simulink model "pfbtest"  (R2015a)
settings: Solver=ode45  StartTime=0.0  StopTime=1500  RelTol=1e-3
libraries: xbsIndex_r4 x275
(part 1 of 2)
settings Model: Creator=tmadden  LastModifiedBy=tmadden
settings OptimizationCC: ExpressionDepthLimit=2147483647
settings DebuggingCC: UnderspecifiedInitializationDetection=Classic  MergeDetectMultiDrivingBlocksExec=none  SolverPrmCheckMsg=warning  StateNameClashWarn=warning

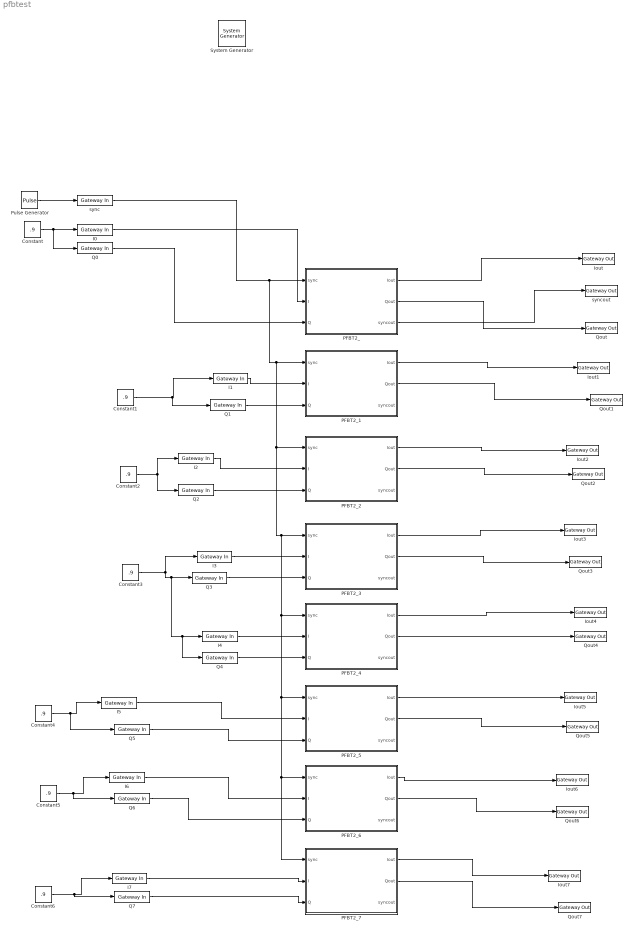
== system pfbtest ==
  " System Generator" : xbsIndex_r4/ System Generator  Tag=genX  xilinxfamily=zynq  part=xc7z100  speed=-2  package=ffv900  synthesis_tool=XST  clock_wrapper=Clock Enables  directory=./untitled/sysgen  proj_type=Project Navigator  Synth_file=XST Defaults  Impl_file=ISE Defaults  testbench=off  simulink_period=1  sysclk_period=10  dcm_input_clock_period=10  incr_netlist=off  trim_vbits=Everywhere in SubSystem  dbl_ovrd=According to Block Masks  core_generation=According to Block Masks  run_coregen=off  deprecated_control=off  eval_field=0  block_type=sysgen
  Constant{,1..6} (7 alike) : Constant  Value=.9
  I{0..7} (8 alike) : xbsIndex_r4/Gateway In  gui_display_data_type=Fixed-point  arith_type="Signed  (2's comp)"  n_bits=18  bin_pt=16  preci_type=Single  exp_width=8  frac_width=24  rows=1  columns=1  quantization="Round  (unbiased: +/- Inf)"  overflow=Saturate  period=1  UseAsADC=off  ADCChannel='1'  interface=None  automatic_assignment=on  address_offset=hex2dec('00')  intf_name=''  intf_description=''  timing_constraint=None  locs_specified=off  LOCs={}  io_standard={}  inherit_from_input=off  hdl_port=on  dbl_ovrd=off  block_type=gatewayin
  Iout{,1..7} (8 alike) : xbsIndex_r4/Gateway Out  inherit_from_input=off  hdl_port=on  rows=1  columns=1  UseAsDAC=off  DACChannel='1'  interface=None  automatic_assignment=on  address_offset=hex2dec('00')  intf_name=''  intf_description=''  timing_constraint=None  locs_specified=off  LOCs={}  io_standard={}  block_type=gatewayout
  PFBT2_ : Subsystem
  PFBT2_1 : Subsystem
  PFBT2_2 : Subsystem
  PFBT2_3 : Subsystem
  PFBT2_4 : Subsystem
  PFBT2_5 : Subsystem
  PFBT2_6 : Subsystem
  PFBT2_7 : Subsystem
  Pulse Generator : DiscretePulseGenerator  Period=1024
  Q{0..7} (8 alike) : xbsIndex_r4/Gateway In  gui_display_data_type=Fixed-point  arith_type="Signed  (2's comp)"  n_bits=18  bin_pt=16  preci_type=Single  exp_width=8  frac_width=24  rows=1  columns=1  quantization="Round  (unbiased: +/- Inf)"  overflow=Saturate  period=1  UseAsADC=off  ADCChannel='1'  interface=None  automatic_assignment=on  address_offset=hex2dec('00')  intf_name=''  intf_description=''  timing_constraint=None  locs_specified=off  LOCs={}  io_standard={}  inherit_from_input=off  hdl_port=on  dbl_ovrd=off  block_type=gatewayin
  Qout{,1..7} (8 alike) : xbsIndex_r4/Gateway Out  inherit_from_input=off  hdl_port=on  rows=1  columns=1  UseAsDAC=off  DACChannel='1'  interface=None  automatic_assignment=on  address_offset=hex2dec('00')  intf_name=''  intf_description=''  timing_constraint=None  locs_specified=off  LOCs={}  io_standard={}  block_type=gatewayout
  sync : xbsIndex_r4/Gateway In  gui_display_data_type=Boolean  arith_type=Boolean  n_bits=16  bin_pt=14  preci_type=Single  exp_width=8  frac_width=24  rows=1  columns=1  quantization="Round  (unbiased: +/- Inf)"  overflow=Saturate  period=1  UseAsADC=off  ADCChannel='1'  interface=None  automatic_assignment=on  address_offset=hex2dec('00')  intf_name=''  intf_description=''  timing_constraint=None  locs_specified=off  LOCs={}  io_standard={}  inherit_from_input=off  hdl_port=on  dbl_ovrd=off  block_type=gatewayin
  syncout : xbsIndex_r4/Gateway Out  inherit_from_input=off  hdl_port=on  rows=1  columns=1  UseAsDAC=off  DACChannel='1'  interface=None  automatic_assignment=on  address_offset=hex2dec('00')  intf_name=''  intf_description=''  timing_constraint=None  locs_specified=off  LOCs={}  io_standard={}  block_type=gatewayout
  wires:
  Pulse Generator/1 -> sync/1
  Constant/1 -> Q0/1, I0/1
  sync/1 -> PFBT2_7/1(sync), PFBT2_6/1(sync), PFBT2_5/1(sync), PFBT2_4/1(sync), PFBT2_3/1(sync), PFBT2_2/1(sync), PFBT2_1/1(sync), PFBT2_/1(sync)
  I0/1 -> PFBT2_/2(I)
  Q0/1 -> PFBT2_/3(Q)
  PFBT2_/1(Iout) -> Iout/1
  PFBT2_/2(Qout) -> Qout/1
  I1/1 -> PFBT2_1/2(I)
  Q1/1 -> PFBT2_1/3(Q)
  I2/1 -> PFBT2_2/2(I)
  Q2/1 -> PFBT2_2/3(Q)
  I3/1 -> PFBT2_3/2(I)
  Q3/1 -> PFBT2_3/3(Q)
  I4/1 -> PFBT2_4/2(I)
  Q4/1 -> PFBT2_4/3(Q)
  I5/1 -> PFBT2_5/2(I)
  Q5/1 -> PFBT2_5/3(Q)
  I6/1 -> PFBT2_6/2(I)
  Q6/1 -> PFBT2_6/3(Q)
  I7/1 -> PFBT2_7/2(I)
  Q7/1 -> PFBT2_7/3(Q)
  Constant6/1 -> Q7/1, I7/1
  Constant5/1 -> Q6/1, I6/1
  Constant4/1 -> Q5/1, I5/1
  Constant3/1 -> Q4/1, I4/1, Q3/1, I3/1
  Constant1/1 -> Q1/1, I1/1
  Constant2/1 -> Q2/1, I2/1
  PFBT2_/3(syncout) -> syncout/1
  PFBT2_1/1(Iout) -> Iout1/1
  PFBT2_1/2(Qout) -> Qout1/1
  PFBT2_2/1(Iout) -> Iout2/1
  PFBT2_2/2(Qout) -> Qout2/1
  PFBT2_3/1(Iout) -> Iout3/1
  PFBT2_3/2(Qout) -> Qout3/1
  PFBT2_4/1(Iout) -> Iout4/1
  PFBT2_4/2(Qout) -> Qout4/1
  PFBT2_5/1(Iout) -> Iout5/1
  PFBT2_5/2(Qout) -> Qout5/1
  PFBT2_6/1(Iout) -> Iout6/1
  PFBT2_6/2(Qout) -> Qout6/1
  PFBT2_7/1(Iout) -> Iout7/1
  PFBT2_7/2(Qout) -> Qout7/1

== system pfbtest/PFBT2_ ==
  sync : Inport
  I : Inport  Port=2
  Q : Inport  Port=3
  AddSub : xbsIndex_r4/AddSub  mode=Addition  use_carryin=off  use_carryout=off  en=off  latency=1  precision=Full  arith_type=Unsigned  n_bits=16  bin_pt=14  quantization=Truncate  overflow=Wrap  use_behavioral_HDL=off  hw_selection=Fabric  pipelined=off  dbl_ovrd=off  block_type=addsub
  AddSub1 : xbsIndex_r4/AddSub  mode=Addition  use_carryin=off  use_carryout=off  en=off  latency=1  precision=Full  arith_type=Unsigned  n_bits=16  bin_pt=14  quantization=Truncate  overflow=Wrap  use_behavioral_HDL=off  hw_selection=Fabric  pipelined=off  dbl_ovrd=off  block_type=addsub
  CoefAddr_ : Subsystem  mask{FL=1024, NS=8}
      mask prompts: FL "FilterLen (FFT Len)"; NS "NumStreams"
  Delay_ : Subsystem  mask{FL=1024, NS=8}
      mask prompts: FL "FiltLen (FFT Len)"; NS "NumStreams"
  Delay_1 : Subsystem  mask{FL=1024, NS=8}
      mask prompts: FL "FiltLen (FFT Len)"; NS "NumStreams"
  TapIQ_1 : Subsystem  mask{FL=1024, WS=0, NS=8, WT=1, NT=2}
      mask prompts: FL "FilterLen"; WS "WhichStream(0..3)"; NS "NStreams"; WT "WhichTap (0..3)"; NT "NumTaps"
  TapIQ_2 : Subsystem  mask{FL=1024, WS=0, NS=8, WT=0, NT=2}
      mask prompts: FL "FilterLen"; WS "WhichStream(0..3)"; NS "NStreams"; WT "WhichTap (0..3)"; NT "NumTaps"
  Iout : Outport
  Qout : Outport  Port=2
  syncout : Outport  Port=3
  wires:
  TapIQ_1/4(syncout) -> syncout/1
  Delay_/1(Iout) -> TapIQ_1/1(Iin)
  Delay_/2(Qout) -> TapIQ_1/2(Qin)
  TapIQ_2/1(Iout) -> Delay_1/1(Iin)
  TapIQ_1/1(Iout) -> AddSub/2
  Delay_1/1(Iout) -> AddSub/1
  Delay_1/2(Qout) -> AddSub1/1
  TapIQ_1/2(Qout) -> AddSub1/2
  Delay_/3(addrout) -> TapIQ_1/3(coefaddr)
  CoefAddr_/1(Addr) -> Delay_/3(addrin), TapIQ_2/3(coefaddr)
  Q/1 -> CoefAddr_/3(Qin)
  I/1 -> CoefAddr_/2(Iin)
  sync/1 -> CoefAddr_/1(sync)
  CoefAddr_/2(Iout) -> TapIQ_2/1(Iin), Delay_/1(Iin)
  CoefAddr_/3(Qout) -> Delay_/2(Qin), TapIQ_2/2(Qin)
  TapIQ_2/4(syncout) -> Delay_1/4(sync)
  CoefAddr_/4(syncout) -> TapIQ_2/4(sync), Delay_/4(sync)
  Delay_/4(syncout) -> TapIQ_1/4(sync)
  AddSub/1 -> Iout/1
  AddSub1/1 -> Qout/1
  TapIQ_2/2(Qout) -> Delay_1/2(Qin)
  TapIQ_2/3(coefaddrout) -> Delay_1/3(addrin)

== system pfbtest/PFBT2_1 ==
  sync : Inport
  I : Inport  Port=2
  Q : Inport  Port=3
  AddSub : xbsIndex_r4/AddSub  mode=Addition  use_carryin=off  use_carryout=off  en=off  latency=1  precision=Full  arith_type=Unsigned  n_bits=16  bin_pt=14  quantization=Truncate  overflow=Wrap  use_behavioral_HDL=off  hw_selection=Fabric  pipelined=off  dbl_ovrd=off  block_type=addsub
  AddSub1 : xbsIndex_r4/AddSub  mode=Addition  use_carryin=off  use_carryout=off  en=off  latency=1  precision=Full  arith_type=Unsigned  n_bits=16  bin_pt=14  quantization=Truncate  overflow=Wrap  use_behavioral_HDL=off  hw_selection=Fabric  pipelined=off  dbl_ovrd=off  block_type=addsub
  CoefAddr_ : Subsystem  mask{FL=1024, NS=8}
      mask prompts: FL "FilterLen (FFT Len)"; NS "NumStreams"
  Delay_ : Subsystem  mask{FL=1024, NS=8}
      mask prompts: FL "FiltLen (FFT Len)"; NS "NumStreams"
  Delay_1 : Subsystem  mask{FL=1024, NS=8}
      mask prompts: FL "FiltLen (FFT Len)"; NS "NumStreams"
  TapIQ_1 : Subsystem  mask{FL=1024, WS=1, NS=8, WT=1, NT=2}
      mask prompts: FL "FilterLen"; WS "WhichStream(0..3)"; NS "NStreams"; WT "WhichTap (0..3)"; NT "NumTaps"
  TapIQ_2 : Subsystem  mask{FL=1024, WS=1, NS=8, WT=0, NT=2}
      mask prompts: FL "FilterLen"; WS "WhichStream(0..3)"; NS "NStreams"; WT "WhichTap (0..3)"; NT "NumTaps"
  Iout : Outport
  Qout : Outport  Port=2
  syncout : Outport  Port=3
  wires:
  TapIQ_1/4(syncout) -> syncout/1
  Delay_/1(Iout) -> TapIQ_1/1(Iin)
  Delay_/2(Qout) -> TapIQ_1/2(Qin)
  TapIQ_2/1(Iout) -> Delay_1/1(Iin)
  TapIQ_1/1(Iout) -> AddSub/2
  Delay_1/1(Iout) -> AddSub/1
  Delay_1/2(Qout) -> AddSub1/1
  TapIQ_1/2(Qout) -> AddSub1/2
  Delay_/3(addrout) -> TapIQ_1/3(coefaddr)
  CoefAddr_/1(Addr) -> Delay_/3(addrin), TapIQ_2/3(coefaddr)
  Q/1 -> CoefAddr_/3(Qin)
  I/1 -> CoefAddr_/2(Iin)
  sync/1 -> CoefAddr_/1(sync)
  CoefAddr_/2(Iout) -> TapIQ_2/1(Iin), Delay_/1(Iin)
  CoefAddr_/3(Qout) -> Delay_/2(Qin), TapIQ_2/2(Qin)
  TapIQ_2/4(syncout) -> Delay_1/4(sync)
  CoefAddr_/4(syncout) -> TapIQ_2/4(sync), Delay_/4(sync)
  Delay_/4(syncout) -> TapIQ_1/4(sync)
  AddSub/1 -> Iout/1
  AddSub1/1 -> Qout/1
  TapIQ_2/2(Qout) -> Delay_1/2(Qin)
  TapIQ_2/3(coefaddrout) -> Delay_1/3(addrin)

== system pfbtest/PFBT2_2 ==
  sync : Inport
  I : Inport  Port=2
  Q : Inport  Port=3
  AddSub : xbsIndex_r4/AddSub  mode=Addition  use_carryin=off  use_carryout=off  en=off  latency=1  precision=Full  arith_type=Unsigned  n_bits=16  bin_pt=14  quantization=Truncate  overflow=Wrap  use_behavioral_HDL=off  hw_selection=Fabric  pipelined=off  dbl_ovrd=off  block_type=addsub
  AddSub1 : xbsIndex_r4/AddSub  mode=Addition  use_carryin=off  use_carryout=off  en=off  latency=1  precision=Full  arith_type=Unsigned  n_bits=16  bin_pt=14  quantization=Truncate  overflow=Wrap  use_behavioral_HDL=off  hw_selection=Fabric  pipelined=off  dbl_ovrd=off  block_type=addsub
  CoefAddr_ : Subsystem  mask{FL=1024, NS=8}
      mask prompts: FL "FilterLen (FFT Len)"; NS "NumStreams"
  Delay_ : Subsystem  mask{FL=512, NS=2}
      mask prompts: FL "FiltLen (FFT Len)"; NS "NumStreams"
  Delay_1 : Subsystem  mask{FL=1024, NS=8}
      mask prompts: FL "FiltLen (FFT Len)"; NS "NumStreams"
  TapIQ_1 : Subsystem  mask{FL=1024, WS=2, NS=8, WT=1, NT=2}
      mask prompts: FL "FilterLen"; WS "WhichStream(0..3)"; NS "NStreams"; WT "WhichTap (0..3)"; NT "NumTaps"
  TapIQ_2 : Subsystem  mask{FL=1024, WS=2, NS=8, WT=0, NT=2}
      mask prompts: FL "FilterLen"; WS "WhichStream(0..3)"; NS "NStreams"; WT "WhichTap (0..3)"; NT "NumTaps"
  Iout : Outport
  Qout : Outport  Port=2
  syncout : Outport  Port=3
  wires:
  TapIQ_1/4(syncout) -> syncout/1
  Delay_/1(Iout) -> TapIQ_1/1(Iin)
  Delay_/2(Qout) -> TapIQ_1/2(Qin)
  TapIQ_2/1(Iout) -> Delay_1/1(Iin)
  TapIQ_1/1(Iout) -> AddSub/2
  Delay_1/1(Iout) -> AddSub/1
  Delay_1/2(Qout) -> AddSub1/1
  TapIQ_1/2(Qout) -> AddSub1/2
  Delay_/3(addrout) -> TapIQ_1/3(coefaddr)
  CoefAddr_/1(Addr) -> Delay_/3(addrin), TapIQ_2/3(coefaddr)
  Q/1 -> CoefAddr_/3(Qin)
  I/1 -> CoefAddr_/2(Iin)
  sync/1 -> CoefAddr_/1(sync)
  CoefAddr_/2(Iout) -> TapIQ_2/1(Iin), Delay_/1(Iin)
  CoefAddr_/3(Qout) -> Delay_/2(Qin), TapIQ_2/2(Qin)
  TapIQ_2/4(syncout) -> Delay_1/4(sync)
  CoefAddr_/4(syncout) -> TapIQ_2/4(sync), Delay_/4(sync)
  Delay_/4(syncout) -> TapIQ_1/4(sync)
  AddSub/1 -> Iout/1
  AddSub1/1 -> Qout/1
  TapIQ_2/2(Qout) -> Delay_1/2(Qin)
  TapIQ_2/3(coefaddrout) -> Delay_1/3(addrin)

== system pfbtest/PFBT2_3 ==
  sync : Inport
  I : Inport  Port=2
  Q : Inport  Port=3
  AddSub : xbsIndex_r4/AddSub  mode=Addition  use_carryin=off  use_carryout=off  en=off  latency=1  precision=Full  arith_type=Unsigned  n_bits=16  bin_pt=14  quantization=Truncate  overflow=Wrap  use_behavioral_HDL=off  hw_selection=Fabric  pipelined=off  dbl_ovrd=off  block_type=addsub
  AddSub1 : xbsIndex_r4/AddSub  mode=Addition  use_carryin=off  use_carryout=off  en=off  latency=1  precision=Full  arith_type=Unsigned  n_bits=16  bin_pt=14  quantization=Truncate  overflow=Wrap  use_behavioral_HDL=off  hw_selection=Fabric  pipelined=off  dbl_ovrd=off  block_type=addsub
  CoefAddr_ : Subsystem  mask{FL=1024, NS=8}
      mask prompts: FL "FilterLen (FFT Len)"; NS "NumStreams"
  Delay_ : Subsystem  mask{FL=1024, NS=8}
      mask prompts: FL "FiltLen (FFT Len)"; NS "NumStreams"
  Delay_1 : Subsystem  mask{FL=1024, NS=8}
      mask prompts: FL "FiltLen (FFT Len)"; NS "NumStreams"
  TapIQ_1 : Subsystem  mask{FL=1024, WS=3, NS=8, WT=1, NT=2}
      mask prompts: FL "FilterLen"; WS "WhichStream(0..3)"; NS "NStreams"; WT "WhichTap (0..3)"; NT "NumTaps"
  TapIQ_2 : Subsystem  mask{FL=1024, WS=3, NS=8, WT=0, NT=2}
      mask prompts: FL "FilterLen"; WS "WhichStream(0..3)"; NS "NStreams"; WT "WhichTap (0..3)"; NT "NumTaps"
  Iout : Outport
  Qout : Outport  Port=2
  syncout : Outport  Port=3
  wires:
  TapIQ_1/4(syncout) -> syncout/1
  Delay_/1(Iout) -> TapIQ_1/1(Iin)
  Delay_/2(Qout) -> TapIQ_1/2(Qin)
  TapIQ_2/1(Iout) -> Delay_1/1(Iin)
  TapIQ_1/1(Iout) -> AddSub/2
  Delay_1/1(Iout) -> AddSub/1
  Delay_1/2(Qout) -> AddSub1/1
  TapIQ_1/2(Qout) -> AddSub1/2
  Delay_/3(addrout) -> TapIQ_1/3(coefaddr)
  CoefAddr_/1(Addr) -> Delay_/3(addrin), TapIQ_2/3(coefaddr)
  Q/1 -> CoefAddr_/3(Qin)
  I/1 -> CoefAddr_/2(Iin)
  sync/1 -> CoefAddr_/1(sync)
  CoefAddr_/2(Iout) -> TapIQ_2/1(Iin), Delay_/1(Iin)
  CoefAddr_/3(Qout) -> Delay_/2(Qin), TapIQ_2/2(Qin)
  TapIQ_2/4(syncout) -> Delay_1/4(sync)
  CoefAddr_/4(syncout) -> TapIQ_2/4(sync), Delay_/4(sync)
  Delay_/4(syncout) -> TapIQ_1/4(sync)
  AddSub/1 -> Iout/1
  AddSub1/1 -> Qout/1
  TapIQ_2/2(Qout) -> Delay_1/2(Qin)
  TapIQ_2/3(coefaddrout) -> Delay_1/3(addrin)

== system pfbtest/PFBT2_4 ==
  sync : Inport
  I : Inport  Port=2
  Q : Inport  Port=3
  AddSub : xbsIndex_r4/AddSub  mode=Addition  use_carryin=off  use_carryout=off  en=off  latency=1  precision=Full  arith_type=Unsigned  n_bits=16  bin_pt=14  quantization=Truncate  overflow=Wrap  use_behavioral_HDL=off  hw_selection=Fabric  pipelined=off  dbl_ovrd=off  block_type=addsub
  AddSub1 : xbsIndex_r4/AddSub  mode=Addition  use_carryin=off  use_carryout=off  en=off  latency=1  precision=Full  arith_type=Unsigned  n_bits=16  bin_pt=14  quantization=Truncate  overflow=Wrap  use_behavioral_HDL=off  hw_selection=Fabric  pipelined=off  dbl_ovrd=off  block_type=addsub
  CoefAddr_ : Subsystem  mask{FL=1024, NS=8}
      mask prompts: FL "FilterLen (FFT Len)"; NS "NumStreams"
  Delay_ : Subsystem  mask{FL=1024, NS=8}
      mask prompts: FL "FiltLen (FFT Len)"; NS "NumStreams"
  Delay_1 : Subsystem  mask{FL=1024, NS=8}
      mask prompts: FL "FiltLen (FFT Len)"; NS "NumStreams"
  TapIQ_1 : Subsystem  mask{FL=1024, WS=4, NS=8, WT=1, NT=2}
      mask prompts: FL "FilterLen"; WS "WhichStream(0..3)"; NS "NStreams"; WT "WhichTap (0..3)"; NT "NumTaps"
  TapIQ_2 : Subsystem  mask{FL=1024, WS=4, NS=8, WT=0, NT=2}
      mask prompts: FL "FilterLen"; WS "WhichStream(0..3)"; NS "NStreams"; WT "WhichTap (0..3)"; NT "NumTaps"
  Iout : Outport
  Qout : Outport  Port=2
  syncout : Outport  Port=3
  wires:
  TapIQ_1/4(syncout) -> syncout/1
  Delay_/1(Iout) -> TapIQ_1/1(Iin)
  Delay_/2(Qout) -> TapIQ_1/2(Qin)
  TapIQ_2/1(Iout) -> Delay_1/1(Iin)
  TapIQ_1/1(Iout) -> AddSub/2
  Delay_1/1(Iout) -> AddSub/1
  Delay_1/2(Qout) -> AddSub1/1
  TapIQ_1/2(Qout) -> AddSub1/2
  Delay_/3(addrout) -> TapIQ_1/3(coefaddr)
  CoefAddr_/1(Addr) -> Delay_/3(addrin), TapIQ_2/3(coefaddr)
  Q/1 -> CoefAddr_/3(Qin)
  I/1 -> CoefAddr_/2(Iin)
  sync/1 -> CoefAddr_/1(sync)
  CoefAddr_/2(Iout) -> TapIQ_2/1(Iin), Delay_/1(Iin)
  CoefAddr_/3(Qout) -> Delay_/2(Qin), TapIQ_2/2(Qin)
  TapIQ_2/4(syncout) -> Delay_1/4(sync)
  CoefAddr_/4(syncout) -> TapIQ_2/4(sync), Delay_/4(sync)
  Delay_/4(syncout) -> TapIQ_1/4(sync)
  AddSub/1 -> Iout/1
  AddSub1/1 -> Qout/1
  TapIQ_2/2(Qout) -> Delay_1/2(Qin)
  TapIQ_2/3(coefaddrout) -> Delay_1/3(addrin)

== system pfbtest/PFBT2_5 ==
  sync : Inport
  I : Inport  Port=2
  Q : Inport  Port=3
  AddSub : xbsIndex_r4/AddSub  mode=Addition  use_carryin=off  use_carryout=off  en=off  latency=1  precision=Full  arith_type=Unsigned  n_bits=16  bin_pt=14  quantization=Truncate  overflow=Wrap  use_behavioral_HDL=off  hw_selection=Fabric  pipelined=off  dbl_ovrd=off  block_type=addsub
  AddSub1 : xbsIndex_r4/AddSub  mode=Addition  use_carryin=off  use_carryout=off  en=off  latency=1  precision=Full  arith_type=Unsigned  n_bits=16  bin_pt=14  quantization=Truncate  overflow=Wrap  use_behavioral_HDL=off  hw_selection=Fabric  pipelined=off  dbl_ovrd=off  block_type=addsub
  CoefAddr_ : Subsystem  mask{FL=1024, NS=8}
      mask prompts: FL "FilterLen (FFT Len)"; NS "NumStreams"
  Delay_ : Subsystem  mask{FL=1024, NS=8}
      mask prompts: FL "FiltLen (FFT Len)"; NS "NumStreams"
  Delay_1 : Subsystem  mask{FL=1024, NS=8}
      mask prompts: FL "FiltLen (FFT Len)"; NS "NumStreams"
  TapIQ_1 : Subsystem  mask{FL=1024, WS=5, NS=8, WT=1, NT=2}
      mask prompts: FL "FilterLen"; WS "WhichStream(0..3)"; NS "NStreams"; WT "WhichTap (0..3)"; NT "NumTaps"
  TapIQ_2 : Subsystem  mask{FL=1024, WS=5, NS=8, WT=0, NT=2}
      mask prompts: FL "FilterLen"; WS "WhichStream(0..3)"; NS "NStreams"; WT "WhichTap (0..3)"; NT "NumTaps"
  Iout : Outport
  Qout : Outport  Port=2
  syncout : Outport  Port=3
  wires:
  TapIQ_1/4(syncout) -> syncout/1
  Delay_/1(Iout) -> TapIQ_1/1(Iin)
  Delay_/2(Qout) -> TapIQ_1/2(Qin)
  TapIQ_2/1(Iout) -> Delay_1/1(Iin)
  TapIQ_1/1(Iout) -> AddSub/2
  Delay_1/1(Iout) -> AddSub/1
  Delay_1/2(Qout) -> AddSub1/1
  TapIQ_1/2(Qout) -> AddSub1/2
  Delay_/3(addrout) -> TapIQ_1/3(coefaddr)
  CoefAddr_/1(Addr) -> Delay_/3(addrin), TapIQ_2/3(coefaddr)
  Q/1 -> CoefAddr_/3(Qin)
  I/1 -> CoefAddr_/2(Iin)
  sync/1 -> CoefAddr_/1(sync)
  CoefAddr_/2(Iout) -> TapIQ_2/1(Iin), Delay_/1(Iin)
  CoefAddr_/3(Qout) -> Delay_/2(Qin), TapIQ_2/2(Qin)
  TapIQ_2/4(syncout) -> Delay_1/4(sync)
  CoefAddr_/4(syncout) -> TapIQ_2/4(sync), Delay_/4(sync)
  Delay_/4(syncout) -> TapIQ_1/4(sync)
  AddSub/1 -> Iout/1
  AddSub1/1 -> Qout/1
  TapIQ_2/2(Qout) -> Delay_1/2(Qin)
  TapIQ_2/3(coefaddrout) -> Delay_1/3(addrin)

== system pfbtest/PFBT2_6 ==
  sync : Inport
  I : Inport  Port=2
  Q : Inport  Port=3
  AddSub : xbsIndex_r4/AddSub  mode=Addition  use_carryin=off  use_carryout=off  en=off  latency=1  precision=Full  arith_type=Unsigned  n_bits=16  bin_pt=14  quantization=Truncate  overflow=Wrap  use_behavioral_HDL=off  hw_selection=Fabric  pipelined=off  dbl_ovrd=off  block_type=addsub
  AddSub1 : xbsIndex_r4/AddSub  mode=Addition  use_carryin=off  use_carryout=off  en=off  latency=1  precision=Full  arith_type=Unsigned  n_bits=16  bin_pt=14  quantization=Truncate  overflow=Wrap  use_behavioral_HDL=off  hw_selection=Fabric  pipelined=off  dbl_ovrd=off  block_type=addsub
  CoefAddr_ : Subsystem  mask{FL=1024, NS=8}
      mask prompts: FL "FilterLen (FFT Len)"; NS "NumStreams"
  Delay_ : Subsystem  mask{FL=1024, NS=8}
      mask prompts: FL "FiltLen (FFT Len)"; NS "NumStreams"
  Delay_1 : Subsystem  mask{FL=1024, NS=8}
      mask prompts: FL "FiltLen (FFT Len)"; NS "NumStreams"
  TapIQ_1 : Subsystem  mask{FL=1024, WS=6, NS=8, WT=1, NT=2}
      mask prompts: FL "FilterLen"; WS "WhichStream(0..3)"; NS "NStreams"; WT "WhichTap (0..3)"; NT "NumTaps"
  TapIQ_2 : Subsystem  mask{FL=1024, WS=6, NS=8, WT=0, NT=2}
      mask prompts: FL "FilterLen"; WS "WhichStream(0..3)"; NS "NStreams"; WT "WhichTap (0..3)"; NT "NumTaps"
  Iout : Outport
  Qout : Outport  Port=2
  syncout : Outport  Port=3
  wires:
  TapIQ_1/4(syncout) -> syncout/1
  Delay_/1(Iout) -> TapIQ_1/1(Iin)
  Delay_/2(Qout) -> TapIQ_1/2(Qin)
  TapIQ_2/1(Iout) -> Delay_1/1(Iin)
  TapIQ_1/1(Iout) -> AddSub/2
  Delay_1/1(Iout) -> AddSub/1
  Delay_1/2(Qout) -> AddSub1/1
  TapIQ_1/2(Qout) -> AddSub1/2
  Delay_/3(addrout) -> TapIQ_1/3(coefaddr)
  CoefAddr_/1(Addr) -> Delay_/3(addrin), TapIQ_2/3(coefaddr)
  Q/1 -> CoefAddr_/3(Qin)
  I/1 -> CoefAddr_/2(Iin)
  sync/1 -> CoefAddr_/1(sync)
  CoefAddr_/2(Iout) -> TapIQ_2/1(Iin), Delay_/1(Iin)
  CoefAddr_/3(Qout) -> Delay_/2(Qin), TapIQ_2/2(Qin)
  TapIQ_2/4(syncout) -> Delay_1/4(sync)
  CoefAddr_/4(syncout) -> TapIQ_2/4(sync), Delay_/4(sync)
  Delay_/4(syncout) -> TapIQ_1/4(sync)
  AddSub/1 -> Iout/1
  AddSub1/1 -> Qout/1
  TapIQ_2/2(Qout) -> Delay_1/2(Qin)
  TapIQ_2/3(coefaddrout) -> Delay_1/3(addrin)

== system pfbtest/PFBT2_7 ==
  sync : Inport
  I : Inport  Port=2
  Q : Inport  Port=3
  AddSub : xbsIndex_r4/AddSub  mode=Addition  use_carryin=off  use_carryout=off  en=off  latency=1  precision=Full  arith_type=Unsigned  n_bits=16  bin_pt=14  quantization=Truncate  overflow=Wrap  use_behavioral_HDL=off  hw_selection=Fabric  pipelined=off  dbl_ovrd=off  block_type=addsub
  AddSub1 : xbsIndex_r4/AddSub  mode=Addition  use_carryin=off  use_carryout=off  en=off  latency=1  precision=Full  arith_type=Unsigned  n_bits=16  bin_pt=14  quantization=Truncate  overflow=Wrap  use_behavioral_HDL=off  hw_selection=Fabric  pipelined=off  dbl_ovrd=off  block_type=addsub
  CoefAddr_ : Subsystem  mask{FL=1024, NS=8}
      mask prompts: FL "FilterLen (FFT Len)"; NS "NumStreams"
  Delay_ : Subsystem  mask{FL=1024, NS=8}
      mask prompts: FL "FiltLen (FFT Len)"; NS "NumStreams"
  Delay_1 : Subsystem  mask{FL=1024, NS=8}
      mask prompts: FL "FiltLen (FFT Len)"; NS "NumStreams"
  TapIQ_1 : Subsystem  mask{FL=1024, WS=7, NS=8, WT=1, NT=2}
      mask prompts: FL "FilterLen"; WS "WhichStream(0..3)"; NS "NStreams"; WT "WhichTap (0..3)"; NT "NumTaps"
  TapIQ_2 : Subsystem  mask{FL=1024, WS=7, NS=8, WT=0, NT=2}
      mask prompts: FL "FilterLen"; WS "WhichStream(0..3)"; NS "NStreams"; WT "WhichTap (0..3)"; NT "NumTaps"
  Iout : Outport
  Qout : Outport  Port=2
  syncout : Outport  Port=3
  wires:
  TapIQ_1/4(syncout) -> syncout/1
  Delay_/1(Iout) -> TapIQ_1/1(Iin)
  Delay_/2(Qout) -> TapIQ_1/2(Qin)
  TapIQ_2/1(Iout) -> Delay_1/1(Iin)
  TapIQ_1/1(Iout) -> AddSub/2
  Delay_1/1(Iout) -> AddSub/1
  Delay_1/2(Qout) -> AddSub1/1
  TapIQ_1/2(Qout) -> AddSub1/2
  Delay_/3(addrout) -> TapIQ_1/3(coefaddr)
  CoefAddr_/1(Addr) -> Delay_/3(addrin), TapIQ_2/3(coefaddr)
  Q/1 -> CoefAddr_/3(Qin)
  I/1 -> CoefAddr_/2(Iin)
  sync/1 -> CoefAddr_/1(sync)
  CoefAddr_/2(Iout) -> TapIQ_2/1(Iin), Delay_/1(Iin)
  CoefAddr_/3(Qout) -> Delay_/2(Qin), TapIQ_2/2(Qin)
  TapIQ_2/4(syncout) -> Delay_1/4(sync)
  CoefAddr_/4(syncout) -> TapIQ_2/4(sync), Delay_/4(sync)
  Delay_/4(syncout) -> TapIQ_1/4(sync)
  AddSub/1 -> Iout/1
  AddSub1/1 -> Qout/1
  TapIQ_2/2(Qout) -> Delay_1/2(Qin)
  TapIQ_2/3(coefaddrout) -> Delay_1/3(addrin)

== system pfbtest/PFBT2_/CoefAddr_ ==
  sync : Inport
  Iin : Inport  Port=2
  Qin : Inport  Port=3
  Counter : xbsIndex_r4/Counter  cnt_type=Free Running  cnt_to=Inf  operation=Up  start_count=0  cnt_by_val=1  arith_type=Unsigned  n_bits=log2(FL/NS)  bin_pt=0  load_pin=off  rst=on  en=off  explicit_period=on  period=1  use_behavioral_HDL=off  implementation=Fabric  dbl_ovrd=off  block_type=counter
  Delay : xbsIndex_r4/Delay  rst=off  infoeditControl=Selection of Reset will increase slice count due to use of real FFs and instead of SRLs  en=off  latency=1  reg_retiming=off  dbl_ovrd=off  block_type=delay
  Delay1 : xbsIndex_r4/Delay  rst=off  infoeditControl=Selection of Reset will increase slice count due to use of real FFs and instead of SRLs  en=off  latency=1  reg_retiming=off  dbl_ovrd=off  block_type=delay
  Delay2 : xbsIndex_r4/Delay  rst=off  infoeditControl=Selection of Reset will increase slice count due to use of real FFs and instead of SRLs  en=off  latency=1  reg_retiming=off  dbl_ovrd=off  block_type=delay
  Addr : Outport
  Iout : Outport  Port=2
  Qout : Outport  Port=3
  syncout : Outport  Port=4
  wires:
  Counter/1 -> Addr/1
  sync/1 -> Delay2/1, Counter/1
  Iin/1 -> Delay/1
  Qin/1 -> Delay1/1
  Delay/1 -> Iout/1
  Delay1/1 -> Qout/1
  Delay2/1 -> syncout/1

== system pfbtest/PFBT2_/Delay_ ==
  Iin : Inport
  Qin : Inport  Port=2
  addrin : Inport  Port=3
  sync : Inport  Port=4
  Delay{,1..3} (4 alike) : xbsIndex_r4/Delay  rst=off  infoeditControl=Selection of Reset will increase slice count due to use of real FFs and instead of SRLs  en=off  latency=FL/NS  reg_retiming=off  dbl_ovrd=off  block_type=delay
  Iout : Outport
  Qout : Outport  Port=2
  addrout : Outport  Port=3
  syncout : Outport  Port=4
  wires:
  Iin/1 -> Delay/1
  Delay/1 -> Iout/1
  Delay1/1 -> Qout/1
  Qin/1 -> Delay1/1
  Delay2/1 -> addrout/1
  addrin/1 -> Delay2/1
  Delay3/1 -> syncout/1
  sync/1 -> Delay3/1

== system pfbtest/PFBT2_/Delay_1 ==
  Iin : Inport
  Qin : Inport  Port=2
  addrin : Inport  Port=3
  sync : Inport  Port=4
  Delay{,1..3} (4 alike) : xbsIndex_r4/Delay  rst=off  infoeditControl=Selection of Reset will increase slice count due to use of real FFs and instead of SRLs  en=off  latency=FL/NS  reg_retiming=off  dbl_ovrd=off  block_type=delay
  Iout : Outport
  Qout : Outport  Port=2
  addrout : Outport  Port=3
  syncout : Outport  Port=4
  wires:
  Iin/1 -> Delay/1
  Delay/1 -> Iout/1
  Delay1/1 -> Qout/1
  Qin/1 -> Delay1/1
  Delay2/1 -> addrout/1
  addrin/1 -> Delay2/1
  Delay3/1 -> syncout/1
  sync/1 -> Delay3/1

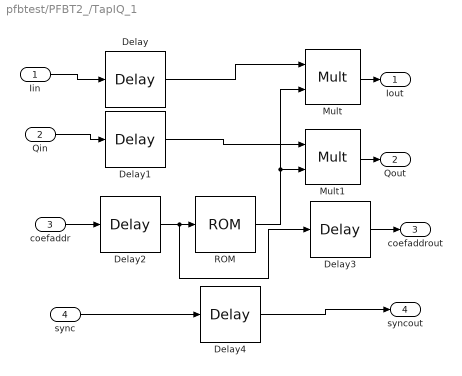
== system pfbtest/PFBT2_/TapIQ_1 ==
  Iin : Inport
  Qin : Inport  Port=2
  coefaddr : Inport  Port=3
  sync : Inport  Port=4
  Delay : xbsIndex_r4/Delay  rst=off  infoeditControl=Selection of Reset will increase slice count due to use of real FFs and instead of SRLs  en=off  latency=FL/NS - 3  reg_retiming=off  dbl_ovrd=off  block_type=delay
  Delay1 : xbsIndex_r4/Delay  rst=off  infoeditControl=Selection of Reset will increase slice count due to use of real FFs and instead of SRLs  en=off  latency=FL/NS -3  reg_retiming=off  dbl_ovrd=off  block_type=delay
  Delay2 : xbsIndex_r4/Delay  rst=off  infoeditControl=Selection of Reset will increase slice count due to use of real FFs and instead of SRLs  en=off  latency=FL/NS -4  reg_retiming=off  dbl_ovrd=off  block_type=delay
  Delay3 : xbsIndex_r4/Delay  rst=off  infoeditControl=Selection of Reset will increase slice count due to use of real FFs and instead of SRLs  en=off  latency=4  reg_retiming=off  dbl_ovrd=off  block_type=delay
  Delay4 : xbsIndex_r4/Delay  rst=off  infoeditControl=Selection of Reset will increase slice count due to use of real FFs and instead of SRLs  en=off  latency=FL/NS  reg_retiming=off  dbl_ovrd=off  block_type=delay
  Mult : xbsIndex_r4/Mult  precision=User Defined  arith_type="Signed  (2's comp)"  n_bits=18  bin_pt=16  quantization=Truncate  overflow=Wrap  en=off  latency=3  use_behavioral_HDL=off  opt=Speed  use_embedded=on  optimum_pipeline=off  pipeline=on  dbl_ovrd=off  use_rpm=on  placement_style=Triangular  block_type=mult
  Mult1 : xbsIndex_r4/Mult  precision=User Defined  arith_type="Signed  (2's comp)"  n_bits=18  bin_pt=16  quantization=Truncate  overflow=Wrap  en=off  latency=3  use_behavioral_HDL=off  opt=Speed  use_embedded=on  optimum_pipeline=off  pipeline=on  dbl_ovrd=off  use_rpm=on  placement_style=Triangular  block_type=mult
  ROM : xbsIndex_r4/ROM  depth=FL/NS  initVector="0.5 - 0.5*cos((2*pi * WT/NT) +  (2*pi/NT)*(WS:NS:(FL-1))/FL)"  distributed_mem=Block RAM  rst=off  init_reg=0  en=off  latency=1  gui_display_data_type=Fixed-point  arith_type="Signed  (2's comp)"  n_bits=18  bin_pt=16  preci_type=Single  exp_width=8  frac_width=24  optimize=Area  use_rpm=on  dbl_ovrd=off  block_type=sprom
  Iout : Outport
  Qout : Outport  Port=2
  coefaddrout : Outport  Port=3
  syncout : Outport  Port=4
  wires:
  Qin/1 -> Delay1/1
  ROM/1 -> Mult1/2, Mult/2
  Mult/1 -> Iout/1
  coefaddr/1 -> Delay2/1
  Mult1/1 -> Qout/1
  Iin/1 -> Delay/1
  Delay/1 -> Mult/1
  Delay1/1 -> Mult1/1
  Delay2/1 -> Delay3/1, ROM/1
  Delay3/1 -> coefaddrout/1
  sync/1 -> Delay4/1
  Delay4/1 -> syncout/1

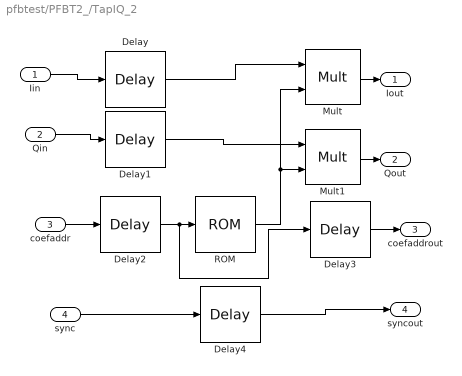
== system pfbtest/PFBT2_/TapIQ_2 ==
  Iin : Inport
  Qin : Inport  Port=2
  coefaddr : Inport  Port=3
  sync : Inport  Port=4
  Delay : xbsIndex_r4/Delay  rst=off  infoeditControl=Selection of Reset will increase slice count due to use of real FFs and instead of SRLs  en=off  latency=FL/NS - 3  reg_retiming=off  dbl_ovrd=off  block_type=delay
  Delay1 : xbsIndex_r4/Delay  rst=off  infoeditControl=Selection of Reset will increase slice count due to use of real FFs and instead of SRLs  en=off  latency=FL/NS -3  reg_retiming=off  dbl_ovrd=off  block_type=delay
  Delay2 : xbsIndex_r4/Delay  rst=off  infoeditControl=Selection of Reset will increase slice count due to use of real FFs and instead of SRLs  en=off  latency=FL/NS -4  reg_retiming=off  dbl_ovrd=off  block_type=delay
  Delay3 : xbsIndex_r4/Delay  rst=off  infoeditControl=Selection of Reset will increase slice count due to use of real FFs and instead of SRLs  en=off  latency=4  reg_retiming=off  dbl_ovrd=off  block_type=delay
  Delay4 : xbsIndex_r4/Delay  rst=off  infoeditControl=Selection of Reset will increase slice count due to use of real FFs and instead of SRLs  en=off  latency=FL/NS  reg_retiming=off  dbl_ovrd=off  block_type=delay
  Mult : xbsIndex_r4/Mult  precision=User Defined  arith_type="Signed  (2's comp)"  n_bits=18  bin_pt=16  quantization=Truncate  overflow=Wrap  en=off  latency=3  use_behavioral_HDL=off  opt=Speed  use_embedded=on  optimum_pipeline=off  pipeline=on  dbl_ovrd=off  use_rpm=on  placement_style=Triangular  block_type=mult
  Mult1 : xbsIndex_r4/Mult  precision=User Defined  arith_type="Signed  (2's comp)"  n_bits=18  bin_pt=16  quantization=Truncate  overflow=Wrap  en=off  latency=3  use_behavioral_HDL=off  opt=Speed  use_embedded=on  optimum_pipeline=off  pipeline=on  dbl_ovrd=off  use_rpm=on  placement_style=Triangular  block_type=mult
  ROM : xbsIndex_r4/ROM  depth=FL/NS  initVector="0.5 - 0.5*cos((2*pi * WT/NT) +  (2*pi/NT)*(WS:NS:(FL-1))/FL)"  distributed_mem=Block RAM  rst=off  init_reg=0  en=off  latency=1  gui_display_data_type=Fixed-point  arith_type="Signed  (2's comp)"  n_bits=18  bin_pt=16  preci_type=Single  exp_width=8  frac_width=24  optimize=Area  use_rpm=on  dbl_ovrd=off  block_type=sprom
  Iout : Outport
  Qout : Outport  Port=2
  coefaddrout : Outport  Port=3
  syncout : Outport  Port=4
  wires:
  Qin/1 -> Delay1/1
  ROM/1 -> Mult1/2, Mult/2
  Mult/1 -> Iout/1
  coefaddr/1 -> Delay2/1
  Mult1/1 -> Qout/1
  Iin/1 -> Delay/1
  Delay/1 -> Mult/1
  Delay1/1 -> Mult1/1
  Delay2/1 -> Delay3/1, ROM/1
  Delay3/1 -> coefaddrout/1
  sync/1 -> Delay4/1
  Delay4/1 -> syncout/1

== system pfbtest/PFBT2_1/CoefAddr_ ==
  sync : Inport
  Iin : Inport  Port=2
  Qin : Inport  Port=3
  Counter : xbsIndex_r4/Counter  cnt_type=Free Running  cnt_to=Inf  operation=Up  start_count=0  cnt_by_val=1  arith_type=Unsigned  n_bits=log2(FL/NS)  bin_pt=0  load_pin=off  rst=on  en=off  explicit_period=on  period=1  use_behavioral_HDL=off  implementation=Fabric  dbl_ovrd=off  block_type=counter
  Delay : xbsIndex_r4/Delay  rst=off  infoeditControl=Selection of Reset will increase slice count due to use of real FFs and instead of SRLs  en=off  latency=1  reg_retiming=off  dbl_ovrd=off  block_type=delay
  Delay1 : xbsIndex_r4/Delay  rst=off  infoeditControl=Selection of Reset will increase slice count due to use of real FFs and instead of SRLs  en=off  latency=1  reg_retiming=off  dbl_ovrd=off  block_type=delay
  Delay2 : xbsIndex_r4/Delay  rst=off  infoeditControl=Selection of Reset will increase slice count due to use of real FFs and instead of SRLs  en=off  latency=1  reg_retiming=off  dbl_ovrd=off  block_type=delay
  Addr : Outport
  Iout : Outport  Port=2
  Qout : Outport  Port=3
  syncout : Outport  Port=4
  wires:
  Counter/1 -> Addr/1
  sync/1 -> Delay2/1, Counter/1
  Iin/1 -> Delay/1
  Qin/1 -> Delay1/1
  Delay/1 -> Iout/1
  Delay1/1 -> Qout/1
  Delay2/1 -> syncout/1

== system pfbtest/PFBT2_1/Delay_ ==
  Iin : Inport
  Qin : Inport  Port=2
  addrin : Inport  Port=3
  sync : Inport  Port=4
  Delay{,1..3} (4 alike) : xbsIndex_r4/Delay  rst=off  infoeditControl=Selection of Reset will increase slice count due to use of real FFs and instead of SRLs  en=off  latency=FL/NS  reg_retiming=off  dbl_ovrd=off  block_type=delay
  Iout : Outport
  Qout : Outport  Port=2
  addrout : Outport  Port=3
  syncout : Outport  Port=4
  wires:
  Iin/1 -> Delay/1
  Delay/1 -> Iout/1
  Delay1/1 -> Qout/1
  Qin/1 -> Delay1/1
  Delay2/1 -> addrout/1
  addrin/1 -> Delay2/1
  Delay3/1 -> syncout/1
  sync/1 -> Delay3/1

== system pfbtest/PFBT2_1/Delay_1 ==
  Iin : Inport
  Qin : Inport  Port=2
  addrin : Inport  Port=3
  sync : Inport  Port=4
  Delay{,1..3} (4 alike) : xbsIndex_r4/Delay  rst=off  infoeditControl=Selection of Reset will increase slice count due to use of real FFs and instead of SRLs  en=off  latency=FL/NS  reg_retiming=off  dbl_ovrd=off  block_type=delay
  Iout : Outport
  Qout : Outport  Port=2
  addrout : Outport  Port=3
  syncout : Outport  Port=4
  wires:
  Iin/1 -> Delay/1
  Delay/1 -> Iout/1
  Delay1/1 -> Qout/1
  Qin/1 -> Delay1/1
  Delay2/1 -> addrout/1
  addrin/1 -> Delay2/1
  Delay3/1 -> syncout/1
  sync/1 -> Delay3/1

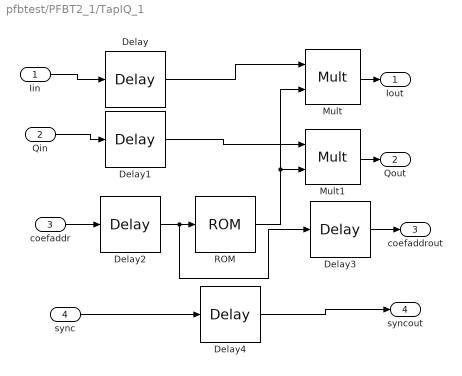
== system pfbtest/PFBT2_1/TapIQ_1 ==
  Iin : Inport
  Qin : Inport  Port=2
  coefaddr : Inport  Port=3
  sync : Inport  Port=4
  Delay : xbsIndex_r4/Delay  rst=off  infoeditControl=Selection of Reset will increase slice count due to use of real FFs and instead of SRLs  en=off  latency=FL/NS - 3  reg_retiming=off  dbl_ovrd=off  block_type=delay
  Delay1 : xbsIndex_r4/Delay  rst=off  infoeditControl=Selection of Reset will increase slice count due to use of real FFs and instead of SRLs  en=off  latency=FL/NS -3  reg_retiming=off  dbl_ovrd=off  block_type=delay
  Delay2 : xbsIndex_r4/Delay  rst=off  infoeditControl=Selection of Reset will increase slice count due to use of real FFs and instead of SRLs  en=off  latency=FL/NS -4  reg_retiming=off  dbl_ovrd=off  block_type=delay
  Delay3 : xbsIndex_r4/Delay  rst=off  infoeditControl=Selection of Reset will increase slice count due to use of real FFs and instead of SRLs  en=off  latency=4  reg_retiming=off  dbl_ovrd=off  block_type=delay
  Delay4 : xbsIndex_r4/Delay  rst=off  infoeditControl=Selection of Reset will increase slice count due to use of real FFs and instead of SRLs  en=off  latency=FL/NS  reg_retiming=off  dbl_ovrd=off  block_type=delay
  Mult : xbsIndex_r4/Mult  precision=User Defined  arith_type="Signed  (2's comp)"  n_bits=18  bin_pt=16  quantization=Truncate  overflow=Wrap  en=off  latency=3  use_behavioral_HDL=off  opt=Speed  use_embedded=on  optimum_pipeline=off  pipeline=on  dbl_ovrd=off  use_rpm=on  placement_style=Triangular  block_type=mult
  Mult1 : xbsIndex_r4/Mult  precision=User Defined  arith_type="Signed  (2's comp)"  n_bits=18  bin_pt=16  quantization=Truncate  overflow=Wrap  en=off  latency=3  use_behavioral_HDL=off  opt=Speed  use_embedded=on  optimum_pipeline=off  pipeline=on  dbl_ovrd=off  use_rpm=on  placement_style=Triangular  block_type=mult
  ROM : xbsIndex_r4/ROM  depth=FL/NS  initVector="0.5 - 0.5*cos((2*pi * WT/NT) +  (2*pi/NT)*(WS:NS:(FL-1))/FL)"  distributed_mem=Block RAM  rst=off  init_reg=0  en=off  latency=1  gui_display_data_type=Fixed-point  arith_type="Signed  (2's comp)"  n_bits=18  bin_pt=16  preci_type=Single  exp_width=8  frac_width=24  optimize=Area  use_rpm=on  dbl_ovrd=off  block_type=sprom
  Iout : Outport
  Qout : Outport  Port=2
  coefaddrout : Outport  Port=3
  syncout : Outport  Port=4
  wires:
  Qin/1 -> Delay1/1
  ROM/1 -> Mult1/2, Mult/2
  Mult/1 -> Iout/1
  coefaddr/1 -> Delay2/1
  Mult1/1 -> Qout/1
  Iin/1 -> Delay/1
  Delay/1 -> Mult/1
  Delay1/1 -> Mult1/1
  Delay2/1 -> Delay3/1, ROM/1
  Delay3/1 -> coefaddrout/1
  sync/1 -> Delay4/1
  Delay4/1 -> syncout/1

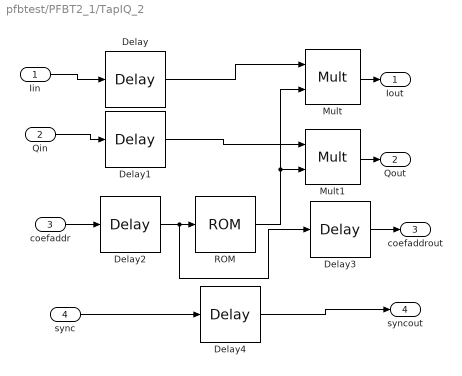
== system pfbtest/PFBT2_1/TapIQ_2 ==
  Iin : Inport
  Qin : Inport  Port=2
  coefaddr : Inport  Port=3
  sync : Inport  Port=4
  Delay : xbsIndex_r4/Delay  rst=off  infoeditControl=Selection of Reset will increase slice count due to use of real FFs and instead of SRLs  en=off  latency=FL/NS - 3  reg_retiming=off  dbl_ovrd=off  block_type=delay
  Delay1 : xbsIndex_r4/Delay  rst=off  infoeditControl=Selection of Reset will increase slice count due to use of real FFs and instead of SRLs  en=off  latency=FL/NS -3  reg_retiming=off  dbl_ovrd=off  block_type=delay
  Delay2 : xbsIndex_r4/Delay  rst=off  infoeditControl=Selection of Reset will increase slice count due to use of real FFs and instead of SRLs  en=off  latency=FL/NS -4  reg_retiming=off  dbl_ovrd=off  block_type=delay
  Delay3 : xbsIndex_r4/Delay  rst=off  infoeditControl=Selection of Reset will increase slice count due to use of real FFs and instead of SRLs  en=off  latency=4  reg_retiming=off  dbl_ovrd=off  block_type=delay
  Delay4 : xbsIndex_r4/Delay  rst=off  infoeditControl=Selection of Reset will increase slice count due to use of real FFs and instead of SRLs  en=off  latency=FL/NS  reg_retiming=off  dbl_ovrd=off  block_type=delay
  Mult : xbsIndex_r4/Mult  precision=User Defined  arith_type="Signed  (2's comp)"  n_bits=18  bin_pt=16  quantization=Truncate  overflow=Wrap  en=off  latency=3  use_behavioral_HDL=off  opt=Speed  use_embedded=on  optimum_pipeline=off  pipeline=on  dbl_ovrd=off  use_rpm=on  placement_style=Triangular  block_type=mult
  Mult1 : xbsIndex_r4/Mult  precision=User Defined  arith_type="Signed  (2's comp)"  n_bits=18  bin_pt=16  quantization=Truncate  overflow=Wrap  en=off  latency=3  use_behavioral_HDL=off  opt=Speed  use_embedded=on  optimum_pipeline=off  pipeline=on  dbl_ovrd=off  use_rpm=on  placement_style=Triangular  block_type=mult
  ROM : xbsIndex_r4/ROM  depth=FL/NS  initVector="0.5 - 0.5*cos((2*pi * WT/NT) +  (2*pi/NT)*(WS:NS:(FL-1))/FL)"  distributed_mem=Block RAM  rst=off  init_reg=0  en=off  latency=1  gui_display_data_type=Fixed-point  arith_type="Signed  (2's comp)"  n_bits=18  bin_pt=16  preci_type=Single  exp_width=8  frac_width=24  optimize=Area  use_rpm=on  dbl_ovrd=off  block_type=sprom
  Iout : Outport
  Qout : Outport  Port=2
  coefaddrout : Outport  Port=3
  syncout : Outport  Port=4
  wires:
  Qin/1 -> Delay1/1
  ROM/1 -> Mult1/2, Mult/2
  Mult/1 -> Iout/1
  coefaddr/1 -> Delay2/1
  Mult1/1 -> Qout/1
  Iin/1 -> Delay/1
  Delay/1 -> Mult/1
  Delay1/1 -> Mult1/1
  Delay2/1 -> Delay3/1, ROM/1
  Delay3/1 -> coefaddrout/1
  sync/1 -> Delay4/1
  Delay4/1 -> syncout/1

== system pfbtest/PFBT2_2/CoefAddr_ ==
  sync : Inport
  Iin : Inport  Port=2
  Qin : Inport  Port=3
  Counter : xbsIndex_r4/Counter  cnt_type=Free Running  cnt_to=Inf  operation=Up  start_count=0  cnt_by_val=1  arith_type=Unsigned  n_bits=log2(FL/NS)  bin_pt=0  load_pin=off  rst=on  en=off  explicit_period=on  period=1  use_behavioral_HDL=off  implementation=Fabric  dbl_ovrd=off  block_type=counter
  Delay : xbsIndex_r4/Delay  rst=off  infoeditControl=Selection of Reset will increase slice count due to use of real FFs and instead of SRLs  en=off  latency=1  reg_retiming=off  dbl_ovrd=off  block_type=delay
  Delay1 : xbsIndex_r4/Delay  rst=off  infoeditControl=Selection of Reset will increase slice count due to use of real FFs and instead of SRLs  en=off  latency=1  reg_retiming=off  dbl_ovrd=off  block_type=delay
  Delay2 : xbsIndex_r4/Delay  rst=off  infoeditControl=Selection of Reset will increase slice count due to use of real FFs and instead of SRLs  en=off  latency=1  reg_retiming=off  dbl_ovrd=off  block_type=delay
  Addr : Outport
  Iout : Outport  Port=2
  Qout : Outport  Port=3
  syncout : Outport  Port=4
  wires:
  Counter/1 -> Addr/1
  sync/1 -> Delay2/1, Counter/1
  Iin/1 -> Delay/1
  Qin/1 -> Delay1/1
  Delay/1 -> Iout/1
  Delay1/1 -> Qout/1
  Delay2/1 -> syncout/1

== system pfbtest/PFBT2_2/Delay_ ==
  Iin : Inport
  Qin : Inport  Port=2
  addrin : Inport  Port=3
  sync : Inport  Port=4
  Delay{,1..3} (4 alike) : xbsIndex_r4/Delay  rst=off  infoeditControl=Selection of Reset will increase slice count due to use of real FFs and instead of SRLs  en=off  latency=FL/NS  reg_retiming=off  dbl_ovrd=off  block_type=delay
  Iout : Outport
  Qout : Outport  Port=2
  addrout : Outport  Port=3
  syncout : Outport  Port=4
  wires:
  Iin/1 -> Delay/1
  Delay/1 -> Iout/1
  Delay1/1 -> Qout/1
  Qin/1 -> Delay1/1
  Delay2/1 -> addrout/1
  addrin/1 -> Delay2/1
  Delay3/1 -> syncout/1
  sync/1 -> Delay3/1

== system pfbtest/PFBT2_2/Delay_1 ==
  Iin : Inport
  Qin : Inport  Port=2
  addrin : Inport  Port=3
  sync : Inport  Port=4
  Delay{,1..3} (4 alike) : xbsIndex_r4/Delay  rst=off  infoeditControl=Selection of Reset will increase slice count due to use of real FFs and instead of SRLs  en=off  latency=FL/NS  reg_retiming=off  dbl_ovrd=off  block_type=delay
  Iout : Outport
  Qout : Outport  Port=2
  addrout : Outport  Port=3
  syncout : Outport  Port=4
  wires:
  Iin/1 -> Delay/1
  Delay/1 -> Iout/1
  Delay1/1 -> Qout/1
  Qin/1 -> Delay1/1
  Delay2/1 -> addrout/1
  addrin/1 -> Delay2/1
  Delay3/1 -> syncout/1
  sync/1 -> Delay3/1

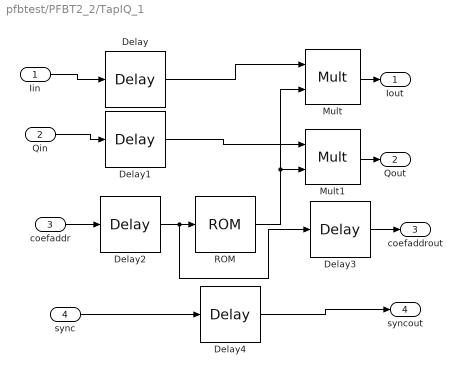
== system pfbtest/PFBT2_2/TapIQ_1 ==
  Iin : Inport
  Qin : Inport  Port=2
  coefaddr : Inport  Port=3
  sync : Inport  Port=4
  Delay : xbsIndex_r4/Delay  rst=off  infoeditControl=Selection of Reset will increase slice count due to use of real FFs and instead of SRLs  en=off  latency=FL/NS - 3  reg_retiming=off  dbl_ovrd=off  block_type=delay
  Delay1 : xbsIndex_r4/Delay  rst=off  infoeditControl=Selection of Reset will increase slice count due to use of real FFs and instead of SRLs  en=off  latency=FL/NS -3  reg_retiming=off  dbl_ovrd=off  block_type=delay
  Delay2 : xbsIndex_r4/Delay  rst=off  infoeditControl=Selection of Reset will increase slice count due to use of real FFs and instead of SRLs  en=off  latency=FL/NS -4  reg_retiming=off  dbl_ovrd=off  block_type=delay
  Delay3 : xbsIndex_r4/Delay  rst=off  infoeditControl=Selection of Reset will increase slice count due to use of real FFs and instead of SRLs  en=off  latency=4  reg_retiming=off  dbl_ovrd=off  block_type=delay
  Delay4 : xbsIndex_r4/Delay  rst=off  infoeditControl=Selection of Reset will increase slice count due to use of real FFs and instead of SRLs  en=off  latency=FL/NS  reg_retiming=off  dbl_ovrd=off  block_type=delay
  Mult : xbsIndex_r4/Mult  precision=User Defined  arith_type="Signed  (2's comp)"  n_bits=18  bin_pt=16  quantization=Truncate  overflow=Wrap  en=off  latency=3  use_behavioral_HDL=off  opt=Speed  use_embedded=on  optimum_pipeline=off  pipeline=on  dbl_ovrd=off  use_rpm=on  placement_style=Triangular  block_type=mult
  Mult1 : xbsIndex_r4/Mult  precision=User Defined  arith_type="Signed  (2's comp)"  n_bits=18  bin_pt=16  quantization=Truncate  overflow=Wrap  en=off  latency=3  use_behavioral_HDL=off  opt=Speed  use_embedded=on  optimum_pipeline=off  pipeline=on  dbl_ovrd=off  use_rpm=on  placement_style=Triangular  block_type=mult
  ROM : xbsIndex_r4/ROM  depth=FL/NS  initVector="0.5 - 0.5*cos((2*pi * WT/NT) +  (2*pi/NT)*(WS:NS:(FL-1))/FL)"  distributed_mem=Block RAM  rst=off  init_reg=0  en=off  latency=1  gui_display_data_type=Fixed-point  arith_type="Signed  (2's comp)"  n_bits=18  bin_pt=16  preci_type=Single  exp_width=8  frac_width=24  optimize=Area  use_rpm=on  dbl_ovrd=off  block_type=sprom
  Iout : Outport
  Qout : Outport  Port=2
  coefaddrout : Outport  Port=3
  syncout : Outport  Port=4
  wires:
  Qin/1 -> Delay1/1
  ROM/1 -> Mult1/2, Mult/2
  Mult/1 -> Iout/1
  coefaddr/1 -> Delay2/1
  Mult1/1 -> Qout/1
  Iin/1 -> Delay/1
  Delay/1 -> Mult/1
  Delay1/1 -> Mult1/1
  Delay2/1 -> Delay3/1, ROM/1
  Delay3/1 -> coefaddrout/1
  sync/1 -> Delay4/1
  Delay4/1 -> syncout/1

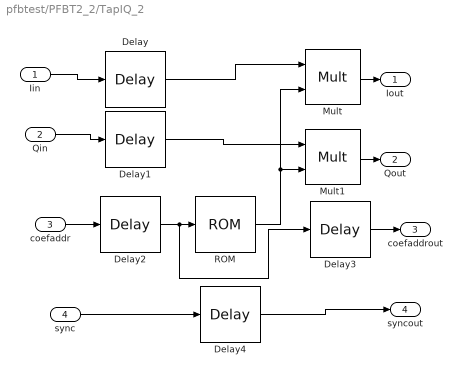
== system pfbtest/PFBT2_2/TapIQ_2 ==
  Iin : Inport
  Qin : Inport  Port=2
  coefaddr : Inport  Port=3
  sync : Inport  Port=4
  Delay : xbsIndex_r4/Delay  rst=off  infoeditControl=Selection of Reset will increase slice count due to use of real FFs and instead of SRLs  en=off  latency=FL/NS - 3  reg_retiming=off  dbl_ovrd=off  block_type=delay
  Delay1 : xbsIndex_r4/Delay  rst=off  infoeditControl=Selection of Reset will increase slice count due to use of real FFs and instead of SRLs  en=off  latency=FL/NS -3  reg_retiming=off  dbl_ovrd=off  block_type=delay
  Delay2 : xbsIndex_r4/Delay  rst=off  infoeditControl=Selection of Reset will increase slice count due to use of real FFs and instead of SRLs  en=off  latency=FL/NS -4  reg_retiming=off  dbl_ovrd=off  block_type=delay
  Delay3 : xbsIndex_r4/Delay  rst=off  infoeditControl=Selection of Reset will increase slice count due to use of real FFs and instead of SRLs  en=off  latency=4  reg_retiming=off  dbl_ovrd=off  block_type=delay
  Delay4 : xbsIndex_r4/Delay  rst=off  infoeditControl=Selection of Reset will increase slice count due to use of real FFs and instead of SRLs  en=off  latency=FL/NS  reg_retiming=off  dbl_ovrd=off  block_type=delay
  Mult : xbsIndex_r4/Mult  precision=User Defined  arith_type="Signed  (2's comp)"  n_bits=18  bin_pt=16  quantization=Truncate  overflow=Wrap  en=off  latency=3  use_behavioral_HDL=off  opt=Speed  use_embedded=on  optimum_pipeline=off  pipeline=on  dbl_ovrd=off  use_rpm=on  placement_style=Triangular  block_type=mult
  Mult1 : xbsIndex_r4/Mult  precision=User Defined  arith_type="Signed  (2's comp)"  n_bits=18  bin_pt=16  quantization=Truncate  overflow=Wrap  en=off  latency=3  use_behavioral_HDL=off  opt=Speed  use_embedded=on  optimum_pipeline=off  pipeline=on  dbl_ovrd=off  use_rpm=on  placement_style=Triangular  block_type=mult
  ROM : xbsIndex_r4/ROM  depth=FL/NS  initVector="0.5 - 0.5*cos((2*pi * WT/NT) +  (2*pi/NT)*(WS:NS:(FL-1))/FL)"  distributed_mem=Block RAM  rst=off  init_reg=0  en=off  latency=1  gui_display_data_type=Fixed-point  arith_type="Signed  (2's comp)"  n_bits=18  bin_pt=16  preci_type=Single  exp_width=8  frac_width=24  optimize=Area  use_rpm=on  dbl_ovrd=off  block_type=sprom
  Iout : Outport
  Qout : Outport  Port=2
  coefaddrout : Outport  Port=3
  syncout : Outport  Port=4
  wires:
  Qin/1 -> Delay1/1
  ROM/1 -> Mult1/2, Mult/2
  Mult/1 -> Iout/1
  coefaddr/1 -> Delay2/1
  Mult1/1 -> Qout/1
  Iin/1 -> Delay/1
  Delay/1 -> Mult/1
  Delay1/1 -> Mult1/1
  Delay2/1 -> Delay3/1, ROM/1
  Delay3/1 -> coefaddrout/1
  sync/1 -> Delay4/1
  Delay4/1 -> syncout/1

== system pfbtest/PFBT2_3/CoefAddr_ ==
  sync : Inport
  Iin : Inport  Port=2
  Qin : Inport  Port=3
  Counter : xbsIndex_r4/Counter  cnt_type=Free Running  cnt_to=Inf  operation=Up  start_count=0  cnt_by_val=1  arith_type=Unsigned  n_bits=log2(FL/NS)  bin_pt=0  load_pin=off  rst=on  en=off  explicit_period=on  period=1  use_behavioral_HDL=off  implementation=Fabric  dbl_ovrd=off  block_type=counter
  Delay : xbsIndex_r4/Delay  rst=off  infoeditControl=Selection of Reset will increase slice count due to use of real FFs and instead of SRLs  en=off  latency=1  reg_retiming=off  dbl_ovrd=off  block_type=delay
  Delay1 : xbsIndex_r4/Delay  rst=off  infoeditControl=Selection of Reset will increase slice count due to use of real FFs and instead of SRLs  en=off  latency=1  reg_retiming=off  dbl_ovrd=off  block_type=delay
  Delay2 : xbsIndex_r4/Delay  rst=off  infoeditControl=Selection of Reset will increase slice count due to use of real FFs and instead of SRLs  en=off  latency=1  reg_retiming=off  dbl_ovrd=off  block_type=delay
  Addr : Outport
  Iout : Outport  Port=2
  Qout : Outport  Port=3
  syncout : Outport  Port=4
  wires:
  Counter/1 -> Addr/1
  sync/1 -> Delay2/1, Counter/1
  Iin/1 -> Delay/1
  Qin/1 -> Delay1/1
  Delay/1 -> Iout/1
  Delay1/1 -> Qout/1
  Delay2/1 -> syncout/1

== system pfbtest/PFBT2_3/Delay_ ==
  Iin : Inport
  Qin : Inport  Port=2
  addrin : Inport  Port=3
  sync : Inport  Port=4
  Delay{,1..3} (4 alike) : xbsIndex_r4/Delay  rst=off  infoeditControl=Selection of Reset will increase slice count due to use of real FFs and instead of SRLs  en=off  latency=FL/NS  reg_retiming=off  dbl_ovrd=off  block_type=delay
  Iout : Outport
  Qout : Outport  Port=2
  addrout : Outport  Port=3
  syncout : Outport  Port=4
  wires:
  Iin/1 -> Delay/1
  Delay/1 -> Iout/1
  Delay1/1 -> Qout/1
  Qin/1 -> Delay1/1
  Delay2/1 -> addrout/1
  addrin/1 -> Delay2/1
  Delay3/1 -> syncout/1
  sync/1 -> Delay3/1

== system pfbtest/PFBT2_3/Delay_1 ==
  Iin : Inport
  Qin : Inport  Port=2
  addrin : Inport  Port=3
  sync : Inport  Port=4
  Delay{,1..3} (4 alike) : xbsIndex_r4/Delay  rst=off  infoeditControl=Selection of Reset will increase slice count due to use of real FFs and instead of SRLs  en=off  latency=FL/NS  reg_retiming=off  dbl_ovrd=off  block_type=delay
  Iout : Outport
  Qout : Outport  Port=2
  addrout : Outport  Port=3
  syncout : Outport  Port=4
  wires:
  Iin/1 -> Delay/1
  Delay/1 -> Iout/1
  Delay1/1 -> Qout/1
  Qin/1 -> Delay1/1
  Delay2/1 -> addrout/1
  addrin/1 -> Delay2/1
  Delay3/1 -> syncout/1
  sync/1 -> Delay3/1
